simulink model "HydraulicSystem"  (R2019a)
settings: Solver=VariableStepAuto  StartTime=0  StopTime=60  RelTol=1e-3
libraries: sh_lib x16, fl_lib x10, nesl_utility x1, sdl_lib x1
settings Model: Creator=Jim  LastModifiedBy=Jim
settings SimscapeCC: SimscapeLogType=all  SimscapeLogLimitData=off

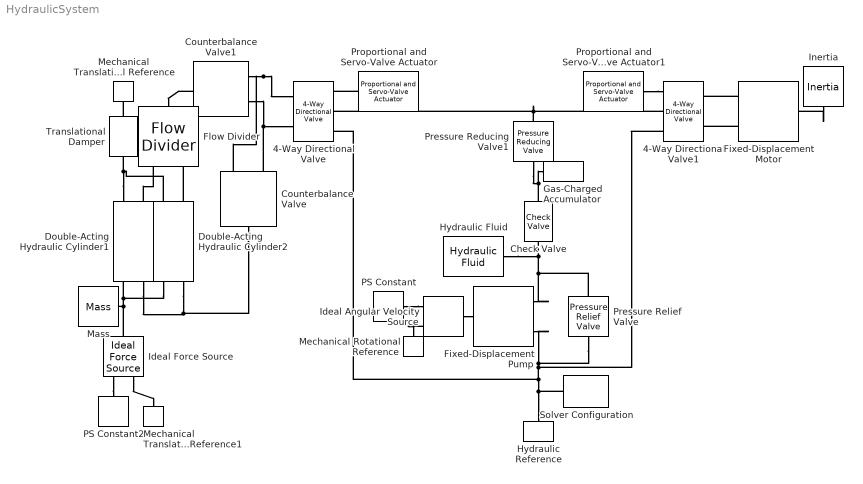
== system HydraulicSystem ==
  4-Way Directional Valve : sh_lib/Valves/Directional Valves/4-Way Directional Valve  area_spec=sh.valves.directional_valves.enum.area_spec.identical  x_0_P_A=0 m  x_0_P_B=0 m  x_0_A_T=0 m  x_0_B_T=0 m  mdl_type_identical=sh.valves.directional_valves.enum.mdl_type.linear  mdl_type_different=sh.valves.directional_valves.enum.mdl_type.linear  opening_max=0.005 m  area_max=0.5e-4 m^2  opening_max_P_A=0.005 m  area_max_P_A=0.5e-4 m^2  opening_max_P_B=0.005 m  area_max_P_B=0.5e-4 m^2  opening_max_A_T=0.005 m  area_max_A_T=0.5e-4 m^2  opening_max_B_T=0.005 m  area_max_B_T=0.5e-4 m^2  opening_area_tab=[-.002, 0, .002, .005, .015] m  area_tab=[1e-09, 2.0352e-07, 4.0736e-05, .00011438, .00034356] m^2  opening_flow_rate_tab=[-.002, 0, .002, .005, .015] m  pressure_tab=[-10000000, -5000000, -2000000, 2000000, 5000000, 10000000] Pa  flow_rate_tab=[-1e-07, -7.0711e-08, -4.4721e-08, 4.4721e-08, 7.0711e-08, 1e-07; -2.0352e-05, -1.4391e-05, -9.1017e-06, 9.1017e-06, 1.4391e-05, 2.0352e-05; -.0040736, -.0028805, -.0018218, .0018218, .0028805, .0040736; -.011438, -.0080879, -.0051152, .0051152, .0080879, .011438; -.034356, -.024293, -.015364, .015364, .024293, .034356] m^3/s  opening_area_tab_P_A=[-.002, 0, .002, .005, .015] m  area_tab_P_A=[1e-09, 2.0352e-07, 4.0736e-05, .00011438, .00034356] m^2  opening_flow_rate_tab_P_A=[-.002, 0, .002, .005, .015] m  pressure_tab_P_A=[-10000000, -5000000, -2000000, 2000000, 5000000, 10000000] Pa  flow_rate_tab_P_A=[-1e-07, -7.0711e-08, -4.4721e-08, 4.4721e-08, 7.0711e-08, 1e-07; -2.0352e-05, -1.4391e-05, -9.1017e-06, 9.1017e-06, 1.4391e-05, 2.0352e-05; -.0040736, -.0028805, -.0018218, .0018218, .0028805, .0040736; -.011438, -.0080879, -.0051152, .0051152, .0080879, .011438; -.034356, -.024293, -.015364, .015364, .024293, .034356] m^3/s  opening_area_tab_P_B=[-.002, 0, .002, .005, .015] m  area_tab_P_B=[1e-09, 2.0352e-07, 4.0736e-05, .00011438, .00034356] m^2  opening_flow_rate_tab_P_B=[-.002, 0, .002, .005, .015] m  pressure_tab_P_B=[-10000000, -5000000, -2000000, 2000000, 5000000, 10000000] Pa  flow_rate_tab_P_B=[-1e-07, -7.0711e-08, -4.4721e-08, 4.4721e-08, 7.0711e-08, 1e-07; -2.0352e-05, -1.4391e-05, -9.1017e-06, 9.1017e-06, 1.4391e-05, 2.0352e-05; -.0040736, -.0028805, -.0018218, .0018218, .0028805, .0040736; -.011438, -.0080879, -.0051152, .0051152, .0080879, .011438; -.034356, -.024293, -.015364, .015364, .024293, .034356] m^3/s  opening_area_tab_A_T=[-.002, 0, .002, .005, .015] m  area_tab_A_T=[1e-09, 2.0352e-07, 4.0736e-05, .00011438, .00034356] m^2  opening_flow_rate_tab_A_T=[-.002, 0, .002, .005, .015] m  pressure_tab_A_T=[-10000000, -5000000, -2000000, 2000000, 5000000, 10000000] Pa  flow_rate_tab_A_T=[-1e-07, -7.0711e-08, -4.4721e-08, 4.4721e-08, 7.0711e-08, 1e-07; -2.0352e-05, -1.4391e-05, -9.1017e-06, 9.1017e-06, 1.4391e-05, 2.0352e-05; -.0040736, -.0028805, -.0018218, .0018218, .0028805, .0040736; -.011438, -.0080879, -.0051152, .0051152, .0080879, .011438; -.034356, -.024293, -.015364, .015364, .024293, .034356] m^3/s  opening_area_tab_B_T=[-.002, 0, .002, .005, .015] m  area_tab_B_T=[1e-09, 2.0352e-07, 4.0736e-05, .00011438, .00034356] m^2  opening_flow_rate_tab_B_T=[-.002, 0, .002, .005, .015] m  pressure_tab_B_T=[-10000000, -5000000, -2000000, 2000000, 5000000, 10000000] Pa  flow_rate_tab_B_T=[-1e-07, -7.0711e-08, -4.4721e-08, 4.4721e-08, 7.0711e-08, 1e-07; -2.0352e-05, -1.4391e-05, -9.1017e-06, 9.1017e-06, 1.4391e-05, 2.0352e-05; -.0040736, -.0028805, -.0018218, .0018218, .0028805, .0040736; -.011438, -.0080879, -.0051152, .0051152, .0080879, .011438; -.034356, -.024293, -.015364, .015364, .024293, .034356] m^3/s  interp_method_identical=sh.valves.directional_valves.enum.interp_method.linear  interp_method_different=sh.valves.directional_valves.enum.interp_method.linear  extrap_method_identical=sh.valves.directional_valves.enum.extrap_method.linear  extrap_method_different=sh.valves.directional_valves.enum.extrap_method.linear  A_leak=1e-12 m^2  C_d=0.7  lam_spec=sh.valves.directional_valves.enum.lam_spec.pressure_ratio  B_lam=0.999  Re_cr=12
      settings: SourceProductName=Simscape Fluids  SourceProductBaseCode=SH
  4-Way Directional Valve1 : sh_lib/Valves/Directional Valves/4-Way Directional Valve  area_spec=sh.valves.directional_valves.enum.area_spec.identical  x_0_P_A=0 m  x_0_P_B=0 m  x_0_A_T=0 m  x_0_B_T=0 m  mdl_type_identical=sh.valves.directional_valves.enum.mdl_type.linear  mdl_type_different=sh.valves.directional_valves.enum.mdl_type.linear  opening_max=0.005 m  area_max=0.5e-4 m^2  opening_max_P_A=0.005 m  area_max_P_A=0.5e-4 m^2  opening_max_P_B=0.005 m  area_max_P_B=0.5e-4 m^2  opening_max_A_T=0.005 m  area_max_A_T=0.5e-4 m^2  opening_max_B_T=0.005 m  area_max_B_T=0.5e-4 m^2  opening_area_tab=[-.002, 0, .002, .005, .015] m  area_tab=[1e-09, 2.0352e-07, 4.0736e-05, .00011438, .00034356] m^2  opening_flow_rate_tab=[-.002, 0, .002, .005, .015] m  pressure_tab=[-10000000, -5000000, -2000000, 2000000, 5000000, 10000000] Pa  flow_rate_tab=[-1e-07, -7.0711e-08, -4.4721e-08, 4.4721e-08, 7.0711e-08, 1e-07; -2.0352e-05, -1.4391e-05, -9.1017e-06, 9.1017e-06, 1.4391e-05, 2.0352e-05; -.0040736, -.0028805, -.0018218, .0018218, .0028805, .0040736; -.011438, -.0080879, -.0051152, .0051152, .0080879, .011438; -.034356, -.024293, -.015364, .015364, .024293, .034356] m^3/s  opening_area_tab_P_A=[-.002, 0, .002, .005, .015] m  area_tab_P_A=[1e-09, 2.0352e-07, 4.0736e-05, .00011438, .00034356] m^2  opening_flow_rate_tab_P_A=[-.002, 0, .002, .005, .015] m  pressure_tab_P_A=[-10000000, -5000000, -2000000, 2000000, 5000000, 10000000] Pa  flow_rate_tab_P_A=[-1e-07, -7.0711e-08, -4.4721e-08, 4.4721e-08, 7.0711e-08, 1e-07; -2.0352e-05, -1.4391e-05, -9.1017e-06, 9.1017e-06, 1.4391e-05, 2.0352e-05; -.0040736, -.0028805, -.0018218, .0018218, .0028805, .0040736; -.011438, -.0080879, -.0051152, .0051152, .0080879, .011438; -.034356, -.024293, -.015364, .015364, .024293, .034356] m^3/s  opening_area_tab_P_B=[-.002, 0, .002, .005, .015] m  area_tab_P_B=[1e-09, 2.0352e-07, 4.0736e-05, .00011438, .00034356] m^2  opening_flow_rate_tab_P_B=[-.002, 0, .002, .005, .015] m  pressure_tab_P_B=[-10000000, -5000000, -2000000, 2000000, 5000000, 10000000] Pa  flow_rate_tab_P_B=[-1e-07, -7.0711e-08, -4.4721e-08, 4.4721e-08, 7.0711e-08, 1e-07; -2.0352e-05, -1.4391e-05, -9.1017e-06, 9.1017e-06, 1.4391e-05, 2.0352e-05; -.0040736, -.0028805, -.0018218, .0018218, .0028805, .0040736; -.011438, -.0080879, -.0051152, .0051152, .0080879, .011438; -.034356, -.024293, -.015364, .015364, .024293, .034356] m^3/s  opening_area_tab_A_T=[-.002, 0, .002, .005, .015] m  area_tab_A_T=[1e-09, 2.0352e-07, 4.0736e-05, .00011438, .00034356] m^2  opening_flow_rate_tab_A_T=[-.002, 0, .002, .005, .015] m  pressure_tab_A_T=[-10000000, -5000000, -2000000, 2000000, 5000000, 10000000] Pa  flow_rate_tab_A_T=[-1e-07, -7.0711e-08, -4.4721e-08, 4.4721e-08, 7.0711e-08, 1e-07; -2.0352e-05, -1.4391e-05, -9.1017e-06, 9.1017e-06, 1.4391e-05, 2.0352e-05; -.0040736, -.0028805, -.0018218, .0018218, .0028805, .0040736; -.011438, -.0080879, -.0051152, .0051152, .0080879, .011438; -.034356, -.024293, -.015364, .015364, .024293, .034356] m^3/s  opening_area_tab_B_T=[-.002, 0, .002, .005, .015] m  area_tab_B_T=[1e-09, 2.0352e-07, 4.0736e-05, .00011438, .00034356] m^2  opening_flow_rate_tab_B_T=[-.002, 0, .002, .005, .015] m  pressure_tab_B_T=[-10000000, -5000000, -2000000, 2000000, 5000000, 10000000] Pa  flow_rate_tab_B_T=[-1e-07, -7.0711e-08, -4.4721e-08, 4.4721e-08, 7.0711e-08, 1e-07; -2.0352e-05, -1.4391e-05, -9.1017e-06, 9.1017e-06, 1.4391e-05, 2.0352e-05; -.0040736, -.0028805, -.0018218, .0018218, .0028805, .0040736; -.011438, -.0080879, -.0051152, .0051152, .0080879, .011438; -.034356, -.024293, -.015364, .015364, .024293, .034356] m^3/s  interp_method_identical=sh.valves.directional_valves.enum.interp_method.linear  interp_method_different=sh.valves.directional_valves.enum.interp_method.linear  extrap_method_identical=sh.valves.directional_valves.enum.extrap_method.linear  extrap_method_different=sh.valves.directional_valves.enum.extrap_method.linear  A_leak=1e-12 m^2  C_d=0.7  lam_spec=sh.valves.directional_valves.enum.lam_spec.pressure_ratio  B_lam=0.999  Re_cr=12
      settings: SourceProductName=Simscape Fluids  SourceProductBaseCode=SH
  Check Valve : sh_lib/Valves/Directional Valves/Check Valve  area_max=1e-4 m^2  pres_crack=300 psi  pres_max=500 psi  C_d=0.7  A_leak=1e-12 m^2  lam_spec=1  B_lam=0.999  Re_cr=12  dynamic=0  tau=0.1 s  area_init=1e-12 m^2
      settings: SourceProductName=Simscape Fluids  SourceProductBaseCode=SH
  Counterbalance Valve : sh_lib/Valves/Flow Control Valves/Counterbalance Valve  pres_set=2000 psi  spring_cp=1e8 Pa/m  p_ratio=3  back_ratio=4  time_const=0.06 s  A_leak=1e-9 m^2  mdl_type=1  or_area_max=8e-5 m^2  or_opening_max=5e-3 m  opening_tab=[-.002, 0, .005, .015] m  area_tab=[1e-09, 4e-09, 1e-05, 1.02e-05] m^2  interp_method=simscape.enum.interpolation.linear  extrap_method=simscape.enum.extrapolation.linear  or_C_d=0.7  or_lam_spec=1  or_B_lam=0.999  or_Re_cr=12  check_area_max=1e-4 m^2  check_pres_crack=0.3e5 Pa  check_pres_max=1.2e5 Pa  check_C_d=0.7  check_lam_spec=1  check_B_lam=0.999  check_Re_cr=12
      settings: SourceProductName=Simscape Fluids  SourceProductBaseCode=SH
  Counterbalance Valve1 : sh_lib/Valves/Flow Control Valves/Counterbalance Valve  pres_set=2000 psi  spring_cp=1e8 Pa/m  p_ratio=3  back_ratio=4  time_const=0.06 s  A_leak=1e-9 m^2  mdl_type=1  or_area_max=8e-5 m^2  or_opening_max=5e-3 m  opening_tab=[-.002, 0, .005, .015] m  area_tab=[1e-09, 4e-09, 1e-05, 1.02e-05] m^2  interp_method=simscape.enum.interpolation.linear  extrap_method=simscape.enum.extrapolation.linear  or_C_d=0.7  or_lam_spec=1  or_B_lam=0.999  or_Re_cr=12  check_area_max=1e-4 m^2  check_pres_crack=0.3e5 Pa  check_pres_max=1.2e5 Pa  check_C_d=0.7  check_lam_spec=1  check_B_lam=0.999  check_Re_cr=12
      settings: SourceProductName=Simscape Fluids  SourceProductBaseCode=SH
  Double-Acting Hydraulic Cylinder1 : sh_lib/Hydraulic Cylinders/Double-Acting Hydraulic Cylinder  area_A=3.14 in^2  area_B=1.91 in^2  stroke=40 in  init_pos=8 in  dead_vol_A=1e-4 m^3  dead_vol_B=1e-4 m^3  init_pressure_A=2000 psi  init_pressure_B=2000 psi  k_sh=1.4  stiff=1e6 N/m  D=150 N/(m/s)  hardstop_model=1  transition=0.1 mm  or=1
      settings: SourceProductName=Simscape Fluids  SourceProductBaseCode=SH
  Double-Acting Hydraulic Cylinder2 : sh_lib/Hydraulic Cylinders/Double-Acting Hydraulic Cylinder  area_A=3.14 in^2  area_B=1.91 in^2  stroke=40 in  init_pos=8 in  dead_vol_A=1e-4 m^3  dead_vol_B=1e-4 m^3  init_pressure_A=2000 psi  init_pressure_B=2000 psi  k_sh=1.4  stiff=1e6 N/m  D=150 N/(m/s)  hardstop_model=1  transition=0.1 mm  or=1
      settings: SourceProductName=Simscape Fluids  SourceProductBaseCode=SH
  Fixed-Displacement Motor : sh_lib/Pumps and Motors/Fixed-Displacement Motor  D=2.2 in^3/rev  loss_spec=1  w_nominal=188 rad/s  pr_nominal=100e5 Pa  visc_nominal=18 cSt  dens_nominal=900 kg/m^3  efficiency_vol=0.92  no_load_torque=0.05 N*m  torque_pressure_coeff=0.6e-6 N*m/Pa  p_diff_eff_TLU=[100000, 1000000, 2000000] Pa  omega_eff_TLU=[25, 50, 100, 200, 300, 400] rad/s  vol_eff_TLU=[.816, .908, .954, .977, .981, .984; .325, .663, .831, .916, .925, .946; .137, .568, .78, .892, .893, .91]  mech_eff_TLU=[.996, .996, .996, .996, .996, .996; .988, .989, .989, .989, .989, .99; .981, .981, .982, .982, .983, .984]  p_diff_loss_TLU=[100000, 1000000, 2000000] Pa  omega_loss_TLU=[25, 50, 100, 200, 300, 400] rad/s  vol_loss_TLU=[.0282, .0253, .0241, .0235, .0291, .0325; .2596, .1271, .1017, .0917, .1216, .1142; .7874, .1901, .141, .1211, .1797, .1978] * 1e-3 m^3/s  mech_loss_TLU=[.002, .002, .002, .002, .002, .002; .06, .055, .055, .055, .055, .05; .19, .19, .18, .18, .17, .16] N*m  pressure_threshold=1e5 Pa  omega_threshold=10 rad/s  quadrant_check=0  pressure_check=0  min_valid_pressure=0 Pa  vol_eff_min=1e-3  vol_eff_max=1  mech_eff_min=1e-3  mech_eff_max=1
      settings: SourceProductName=Simscape Fluids  SourceProductBaseCode=SH
  Fixed-Displacement Pump : sh_lib/Pumps and Motors/Fixed-Displacement Pump  D=0.042 in^3/rev  loss_spec=1  w_nominal=3330 rpm  pr_nominal=3000 psi  visc_nominal=18 cSt  dens_nominal=900 kg/m^3  efficiency_vol=0.92  no_load_torque=0.05 N*m  torque_pressure_coeff=0.6e-6 N*m/Pa  p_diff_eff_TLU=[100000, 1000000, 2000000] Pa  omega_eff_TLU=[25, 50, 100, 200, 300, 400] rad/s  vol_eff_TLU=[.816, .908, .954, .977, .981, .984; .325, .663, .831, .916, .925, .946; .137, .568, .78, .892, .893, .91]  mech_eff_TLU=[.996, .996, .996, .996, .996, .996; .988, .989, .989, .989, .989, .99; .981, .981, .982, .982, .983, .984]  p_diff_loss_TLU=[100000, 1000000, 2000000] Pa  omega_loss_TLU=[25, 50, 100, 200, 300, 400] rad/s  vol_loss_TLU=[.023, .023, .023, .023, .0285, .032; .0844, .0842, .0845, .084, .1125, .108; .1079, .108, .11, .108, .1605, .18] * 1e-3 m^3/s  mech_loss_TLU=[.002, .002, .002, .002, .002, .002; .0607, .0556, .0556, .0556, .0556, .0505; .1937, .1937, .1833, .1833, .1729, .1626] N*m  pressure_threshold=1e5 Pa  omega_threshold=10 rad/s  quadrant_check=0  pressure_check=0  min_valid_pressure=0 Pa  vol_eff_min=1e-3  vol_eff_max=1  mech_eff_min=1e-3  mech_eff_max=1
      settings: SourceProductName=Simscape Fluids  SourceProductBaseCode=SH
  Flow Divider : sh_lib/Valves/Flow Control Valves/Flow Divider  area_A=1e-4 m^2  area_B=1e-4 m^2  C_d_A=0.7  C_d_B=0.7  lam_spec=1  B_lam_A=0.999  B_lam_B=0.999  Re_cr_A=10  Re_cr_B=10  orifice_d=0.005 m  orifice_numb=4  C_d_or=0.65  init_A=0.0025 m  init_B=0.0025 m  leak_area=1e-9 m^2  lam_spec_or=1  B_lam_or_A=0.999  B_lam_or_B=0.999  Re_cr_or_A=10  Re_cr_or_B=10  area_sc=1.6e-4 m^2  stroke=0.005 m  spring_rate=1e3 N/m  damping=150 N/(m/s)  stop_coefficient=1e12 s*N/m^2
      settings: SourceProductName=Simscape Fluids  SourceProductBaseCode=SH
  Gas-Charged Accumulator : sh_lib/Accumulators/Gas-Charged Accumulator  capacity=1 l  dead_volume=0.01 gal  pr_preload=1200 psi  k_sh=1.4  stiff_coeff=1e10 Pa/m^3  penetr_coeff=1e10 s*Pa/m^6  flow_rate_specify=on  flow_rate_priority=None  flow_rate=0 gpm  flow_rate_nominal_specify=off  flow_rate_nominal_unit=m^3/s  flow_rate_nominal_value=1  liquid_volume_specify=on  liquid_volume_priority=High  liquid_volume=0 l  liquid_volume_nominal_specify=off  liquid_volume_nominal_unit=m^3  liquid_volume_nominal_value=1  liquid_pressure_specify=on  liquid_pressure_priority=None  liquid_pressure=0 psi  liquid_pressure_nominal_specify=off  liquid_pressure_nominal_unit=Pa  liquid_pressure_nominal_value=1
      settings: SourceProductName=Simscape Fluids  SourceProductBaseCode=SH
  Hydraulic Fluid : sh_lib/Hydraulic Utilities/Hydraulic Fluid  DataSource=1  SelFluid=1  SysTemp=-20  TrapAir=0.005  ViscDerFactor=1  range_error=2
      settings: SourceProductName=Simscape Fluids
  Hydraulic Reference : fl_lib/Hydraulic/Hydraulic Elements/Hydraulic Reference
      settings: SourceProductName=Simscape
  Ideal Angular Velocity Source : fl_lib/Mechanical/Mechanical Sources/Ideal Angular Velocity Source
  Ideal Force Source : fl_lib/Mechanical/Mechanical Sources/Ideal Force Source
  Inertia : fl_lib/Mechanical/Rotational Elements/Inertia  inertia=100 lbm*ft^2  w_specify=off  w_priority=High  w=0 rad/s  w_nominal_specify=off  w_nominal_unit=rad/s  w_nominal_value=1  t_specify=off  t_priority=None  t=0 N*m  t_nominal_specify=off  t_nominal_unit=N*m  t_nominal_value=1
  Mass : fl_lib/Mechanical/Translational Elements/Mass  mass=1000 lbm  v_specify=off  v_priority=High  v=0 m/s  v_nominal_specify=off  v_nominal_unit=m/s  v_nominal_value=1  f_specify=off  f_priority=None  f=0 N  f_nominal_specify=off  f_nominal_unit=N  f_nominal_value=1
  Mechanical Rotational Reference : fl_lib/Mechanical/Rotational Elements/Mechanical Rotational Reference
  Mechanical Translational Reference : fl_lib/Mechanical/Translational Elements/Mechanical Translational Reference
  Mechanical Translational Reference1 : fl_lib/Mechanical/Translational Elements/Mechanical Translational Reference
  PS Constant : fl_lib/Physical Signals/Sources/PS Constant  constant=3300 rpm
  PS Constant2 : fl_lib/Physical Signals/Sources/PS Constant  constant=-4000 lb
  Pressure Reducing Valve1 : sh_lib/Valves/Pressure Control Valves/Pressure Reducing Valve  valve_area_spec=1  p_diff_TLU=[30.15e5 : 15e3 : 31.35e5] Pa  area_TLU=[9 : -1 : 1] .* 1e-5 m^2  area_max=1e-4 m^2  pres_set=2000 psi  reg_range=1.5e5 Pa  C_d=0.7  A_leak=1e-12 m^2  lam_spec=1  B_lam=0.999  Re_cr=12  dynamic=0  tau=0.1 s  area_init=1e-12 m^2
      settings: SourceProductName=Simscape Fluids  SourceProductBaseCode=SH
  Pressure Relief Valve : sh_lib/Valves/Pressure Control Valves/Pressure Relief Valve  valve_area_spec=1  p_diff_TLU=[30.15e5 : 15e3 : 31.35e5] Pa  area_TLU=[1 : 1 : 9] .* 1e-5 m^2  area_max=1e-4 m^2  pres_set=3300 psi  reg_range=5e5 Pa  C_d=0.7  A_leak=1e-12 m^2  lam_spec=1  B_lam=0.999  Re_cr=12  dynamic=0  tau=0.1 s  area_init=1e-12 m^2
      settings: SourceProductName=Simscape Fluids  SourceProductBaseCode=SH
  Proportional and Servo-Valve Actuator : sh_lib/Valves/Valve Actuators/Proportional and Servo-Valve Actuator  gain=1  time_constant=0.002 s  saturation=0.3
      settings: SourceProductName=Simscape Fluids  SourceProductBaseCode=SH
  Proportional and Servo-Valve Actuator1 : sh_lib/Valves/Valve Actuators/Proportional and Servo-Valve Actuator  gain=1  time_constant=0.002 s  saturation=0.3
      settings: SourceProductName=Simscape Fluids  SourceProductBaseCode=SH
  Solver Configuration : nesl_utility/Solver Configuration  PhysicalDomain=network_engine_domain  SubClassName=solver  LeftPortType=input  RightPortType=generic  Tones=[]  Harmonics=[]  SimulateNoise=off  Profile=off  UseLocalSampling=off  EnableSwitchedLinearOptims=on  FrequencyDomain=off  UseCCode=off  RelTol=0.001  AbsTol=1e-06  MinStep=1e-09  ToWorkspace=off  RevertToSquareIcSolve=off  NumHomotopyIterations=100  PhasorMode=off  PhasorModeNumHarmonics=1  DoDC=off  ResidualTolerance=1e-09  UseLocalSolver=off  LocalSolverChoice=NE_BACKWARD_EULER_ADVANCER  LocalSolverSampleTime=0.001  DoFixedCost=off  MaxNonlinIter=3  MaxModeIter=2  LinearAlgebra=auto  EquationFormulation=NE_TIME_EF  DelaysMemoryBudget=1024  AutomaticFiltering=on  FilteringTimeConstant=0.001  PartitionStorageMethod=AS_NEEDED  PartitionMemoryBudget=1024  PartitionMethod=ROBUST
  Translational Damper : sdl_lib/Couplings & Drives/Springs & Dampers/Translational Damper  D=1 lbf/(ft/s)  enable_faults=0  b_fault=1e6 N/(m/s)  temporal_fault=0  fault_time=5 s  shock_fault=0  acceleration_limit=100 m/s^2  shock_limit=1  report_fault=1
      settings: SourceProductName=Simscape Driveline  SourceProductBaseCode=LD
  connections:
  Ideal Angular Velocity Source/LConn1 -- Fixed-Displacement Pump/LConn1
  Ideal Angular Velocity Source/RConn2 -- Mechanical Rotational Reference/LConn1
  Double-Acting Hydraulic Cylinder1/LConn1 -- Double-Acting Hydraulic Cylinder2/LConn1 -- Translational Damper/LConn1
  Double-Acting Hydraulic Cylinder1/LConn2 -- Flow Divider/RConn1
  Double-Acting Hydraulic Cylinder2/LConn2 -- Flow Divider/RConn2
  Ideal Force Source/LConn1 -- Double-Acting Hydraulic Cylinder2/RConn1 -- Double-Acting Hydraulic Cylinder1/RConn1 -- Mass/LConn1
  Ideal Force Source/RConn2 -- Mechanical Translational Reference1/LConn1
  Fixed-Displacement Motor/LConn1 -- 4-Way Directional Valve1/LConn1
  Inertia/LConn1 -- Fixed-Displacement Motor/RConn1
  Translational Damper/RConn1 -- Mechanical Translational Reference/LConn1
  Ideal Force Source/RConn1 -- PS Constant2/RConn1
  Fixed-Displacement Motor/LConn2 -- 4-Way Directional Valve1/LConn2
  PS Constant/RConn1 -- Ideal Angular Velocity Source/RConn1
  Fixed-Displacement Pump/RConn2 -- 4-Way Directional Valve1/RConn3 -- 4-Way Directional Valve/RConn3 -- Solver Configuration/RConn1 -- Hydraulic Reference/LConn1 -- Pressure Relief Valve/RConn1
  Fixed-Displacement Pump/RConn1 -- Pressure Relief Valve/LConn1 -- Hydraulic Fluid/RConn1 -- Check Valve/LConn1
  Check Valve/RConn1 -- Pressure Reducing Valve1/LConn1 -- Gas-Charged Accumulator/RConn1
  Pressure Reducing Valve1/RConn1 -- 4-Way Directional Valve1/RConn2 -- 4-Way Directional Valve/RConn2
  Double-Acting Hydraulic Cylinder1/RConn2 -- Double-Acting Hydraulic Cylinder2/RConn2 -- Counterbalance Valve/RConn1
  Counterbalance Valve/LConn1 -- Counterbalance Valve1/LConn2 -- 4-Way Directional Valve/LConn2
  Proportional and Servo-Valve Actuator/RConn1 -- 4-Way Directional Valve/RConn1
  Proportional and Servo-Valve Actuator1/RConn1 -- 4-Way Directional Valve1/RConn1
  Counterbalance Valve1/RConn1 -- Flow Divider/LConn1
  Counterbalance Valve1/LConn1 -- Counterbalance Valve/LConn2 -- 4-Way Directional Valve/LConn1
